simulink library "INP_DMP_ManOver"  (R2024b)
settings: Solver=VariableStepAuto  StartTime=0.0  StopTime=10.0  RelTol=1e-3
undefined symbols (not defined in the file): INP_DMP_p_StrkDmpLoLimFrLe_mm, INP_DMP_p_StrkDmpLoLimFrRi_mm, INP_DMP_p_StrkDmpLoLimReLe_mm, INP_DMP_p_StrkDmpLoLimReRi_mm, INP_DMP_p_StrkDmpUpLimFrLe_mm, INP_DMP_p_StrkDmpUpLimFrRi_mm, INP_DMP_p_StrkDmpUpLimReLe_mm, INP_DMP_p_StrkDmpUpLimReRi_mm, INP_DMP_p_SwtStrkDmpFrLe_na, INP_DMP_p_SwtStrkDmpFrRi_na, INP_DMP_p_SwtStrkDmpReLe_na, INP_DMP_p_SwtStrkDmpReRi_na, INP_DMP_s_StrkDmpFrLeMan_mm, INP_DMP_s_StrkDmpFrRiMan_mm, INP_DMP_s_StrkDmpReLeMan_mm, INP_DMP_s_StrkDmpReRiMan_mm, INP_DRVR_p_AngRatStWhlLoLim_radps, INP_DRVR_p_AngRatStWhlUpLim_radps, INP_DRVR_p_AngStWhlLoLim_rad, INP_DRVR_p_AngStWhlUpLim_rad, INP_DRVR_p_PosRatThrLoLim_p100ps, INP_DRVR_p_PosRatThrMan_p100ps, INP_DRVR_p_PosRatThrUpLim_p100ps, INP_DRVR_p_PosThrLoLim_p100, INP_DRVR_p_PosThrMan_p100, INP_DRVR_p_PosThrUpLim_p100, INP_DRVR_p_SwtAngRatStWhlMan_na, INP_DRVR_p_SwtAngStWhlMan_na, INP_DRVR_p_SwtPosRatThrMan_na, INP_DRVR_p_SwtPosThrMan_na, INP_DRVR_s_AngRatStWhlMan_radps, INP_DRVR_s_AngStWhlMan_rad
libraries: simulink x8
settings Model: Creator=blatak  LastModifiedBy=jmbsp

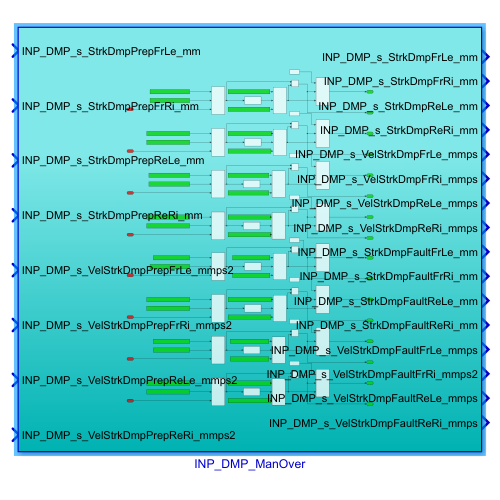
[thumbnail: Simulink's stored preview of the top-level diagram]
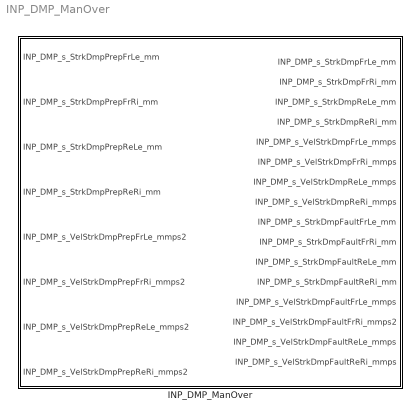
== system INP_DMP_ManOver ==
  INP_DMP_ManOver : Subsystem

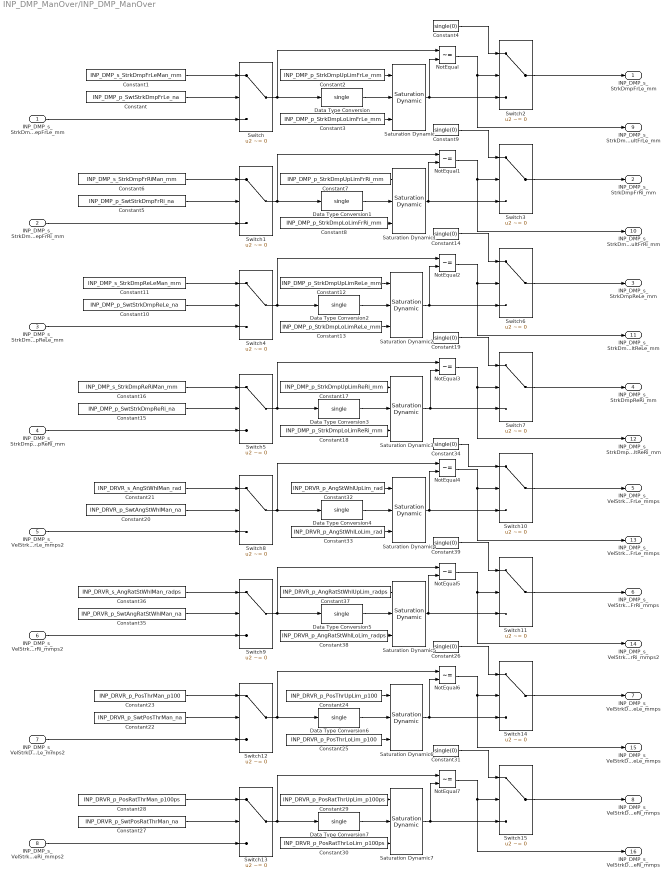
== system INP_DMP_ManOver/INP_DMP_ManOver ==
  INP_DMP_s_StrkDmpPrepFrLe_mm : Inport
  INP_DMP_s_StrkDmpPrepFrRi_mm : Inport  Port=2
  INP_DMP_s_StrkDmpPrepReLe_mm : Inport  Port=3
  INP_DMP_s_StrkDmpPrepReRi_mm : Inport  Port=4
  INP_DMP_s_VelStrkDmpPrepFrLe_mmps2 : Inport  Port=5
  INP_DMP_s_VelStrkDmpPrepFrRi_mmps2 : Inport  Port=6
  INP_DMP_s_VelStrkDmpPrepReLe_mmps2 : Inport  Port=7
  INP_DMP_s_VelStrkDmpPrepReRi_mmps2 : Inport  Port=8
  Constant : Constant  Description=|  Value=INP_DMP_p_SwtStrkDmpFrLe_na
      | Switch for manual override of the longitudinal acceleration value, if 1 instead the measured 
      | value the INP_IMU_p_ALgtVehMan_mps2 is used
  Constant1 : Constant  Description=|  Value=INP_DMP_s_StrkDmpFrLeMan_mm
      | Value for longitudinal acceleration, which is used if the INP_IMU_p_SwtAXxxVehMan_na
      | is set to 1 instead of the measured value
  Constant10 : Constant  Description=|  Value=INP_DMP_p_SwtStrkDmpReLe_na
      | Switch for manual override of the longitudinal acceleration value, if 1 instead the measured 
      | value the INP_IMU_p_ALgtVehMan_mps2 is used
  Constant11 : Constant  Description=|  Value=INP_DMP_s_StrkDmpReLeMan_mm
      | Value for longitudinal acceleration, which is used if the INP_IMU_p_SwtAXxxVehMan_na
      | is set to 1 instead of the measured value
  Constant12 : Constant  Description=Upper saturation limit for longitudinal acceleration  Value=INP_DMP_p_StrkDmpUpLimReLe_mm
  Constant13 : Constant  Description=Lower saturation limit for longitudinal acceleration  Value=INP_DMP_p_StrkDmpLoLimReLe_mm
  Constant{4,9,14,19,26,31,34,39} (8 alike) : Constant  Value=single(0)
  Constant15 : Constant  Description=|  Value=INP_DMP_p_SwtStrkDmpReRi_na
      | Switch for manual override of the longitudinal acceleration value, if 1 instead the measured 
      | value the INP_IMU_p_ALgtVehMan_mps2 is used
  Constant16 : Constant  Description=|  Value=INP_DMP_s_StrkDmpReRiMan_mm
      | Value for longitudinal acceleration, which is used if the INP_IMU_p_SwtAXxxVehMan_na
      | is set to 1 instead of the measured value
  Constant17 : Constant  Description=Upper saturation limit for longitudinal acceleration  Value=INP_DMP_p_StrkDmpUpLimReRi_mm
  Constant18 : Constant  Description=Lower saturation limit for longitudinal acceleration  Value=INP_DMP_p_StrkDmpLoLimReRi_mm
  Constant2 : Constant  Description=Upper saturation limit for longitudinal acceleration  Value=INP_DMP_p_StrkDmpUpLimFrLe_mm
  Constant20 : Constant  Description=|  Value=INP_DRVR_p_SwtAngStWhlMan_na
      | Switch for manual override of the longitudinal acceleration value, if 1 instead the measured 
      | value the INP_IMU_p_ALgtVehMan_mps2 is used
  Constant21 : Constant  Description=|  Value=INP_DRVR_s_AngStWhlMan_rad
      | Value for longitudinal acceleration, which is used if the INP_IMU_p_SwtAXxxVehMan_na
      | is set to 1 instead of the measured value
  Constant22 : Constant  Description=|  Value=INP_DRVR_p_SwtPosThrMan_na
      | Switch for manual override of the longitudinal acceleration value, if 1 instead the measured 
      | value the INP_IMU_p_ALgtVehMan_mps2 is used
  Constant23 : Constant  Description=|  Value=INP_DRVR_p_PosThrMan_p100
      | Value for longitudinal acceleration, which is used if the INP_IMU_p_SwtAXxxVehMan_na
      | is set to 1 instead of the measured value
  Constant24 : Constant  Description=Upper saturation limit for longitudinal acceleration  Value=INP_DRVR_p_PosThrUpLim_p100
  Constant25 : Constant  Description=Lower saturation limit for longitudinal acceleration  Value=INP_DRVR_p_PosThrLoLim_p100
  Constant27 : Constant  Description=|  Value=INP_DRVR_p_SwtPosRatThrMan_na
      | Switch for manual override of the longitudinal acceleration value, if 1 instead the measured 
      | value the INP_IMU_p_ALgtVehMan_mps2 is used
  Constant28 : Constant  Description=|  Value=INP_DRVR_p_PosRatThrMan_p100ps
      | Value for longitudinal acceleration, which is used if the INP_IMU_p_SwtAXxxVehMan_na
      | is set to 1 instead of the measured value
  Constant29 : Constant  Description=Upper saturation limit for longitudinal acceleration  Value=INP_DRVR_p_PosRatThrUpLim_p100ps
  Constant3 : Constant  Description=Lower saturation limit for longitudinal acceleration  Value=INP_DMP_p_StrkDmpLoLimFrLe_mm
  Constant30 : Constant  Description=Lower saturation limit for longitudinal acceleration  Value=INP_DRVR_p_PosRatThrLoLim_p100ps
  Constant32 : Constant  Description=Upper saturation limit for longitudinal acceleration  Value=INP_DRVR_p_AngStWhlUpLim_rad
  Constant33 : Constant  Description=Lower saturation limit for longitudinal acceleration  Value=INP_DRVR_p_AngStWhlLoLim_rad
  Constant35 : Constant  Description=|  Value=INP_DRVR_p_SwtAngRatStWhlMan_na
      | Switch for manual override of the longitudinal acceleration value, if 1 instead the measured 
      | value the INP_IMU_p_ALgtVehMan_mps2 is used
  Constant36 : Constant  Description=|  Value=INP_DRVR_s_AngRatStWhlMan_radps
      | Value for longitudinal acceleration, which is used if the INP_IMU_p_SwtAXxxVehMan_na
      | is set to 1 instead of the measured value
  Constant37 : Constant  Description=Upper saturation limit for longitudinal acceleration  Value=INP_DRVR_p_AngRatStWhlUpLim_radps
  Constant38 : Constant  Description=Lower saturation limit for longitudinal acceleration  Value=INP_DRVR_p_AngRatStWhlLoLim_radps
  Constant5 : Constant  Description=|  Value=INP_DMP_p_SwtStrkDmpFrRi_na
      | Switch for manual override of the longitudinal acceleration value, if 1 instead the measured 
      | value the INP_IMU_p_ALgtVehMan_mps2 is used
  Constant6 : Constant  Description=|  Value=INP_DMP_s_StrkDmpFrRiMan_mm
      | Value for longitudinal acceleration, which is used if the INP_IMU_p_SwtAXxxVehMan_na
      | is set to 1 instead of the measured value
  Constant7 : Constant  Description=Upper saturation limit for longitudinal acceleration  Value=INP_DMP_p_StrkDmpUpLimFrRi_mm
  Constant8 : Constant  Description=Lower saturation limit for longitudinal acceleration  Value=INP_DMP_p_StrkDmpLoLimFrRi_mm
  Data Type Conversion{,1..7} (8 alike) : DataTypeConversion  OutDataTypeStr=single  SaturateOnIntegerOverflow=off  RndMeth=Floor
  NotEqual{,1..7} (8 alike) : RelationalOperator  Operator=~=  OutDataTypeStr=boolean  RndMeth=Simplest  InputSameDT=off
  Saturation Dynamic{,1..7} (8 alike) : simulink/Discontinuities/Saturation Dynamic  OutMin=[]  OutMax=[]  OutDataTypeStr=Inherit: Same as second input  OutDataType=fixdt(1, 16)  OutScaling=2^-10  DoSatur=off
  Switch{,1..15} (16 alike) : Switch  Criteria=u2 ~= 0  SaturateOnIntegerOverflow=off  InputSameDT=off
  INP_DMP_s_StrkDmpFrLe_mm : Outport
  INP_DMP_s_StrkDmpFrRi_mm : Outport  Port=2
  INP_DMP_s_StrkDmpReLe_mm : Outport  Port=3
  INP_DMP_s_StrkDmpReRi_mm : Outport  Port=4
  INP_DMP_s_VelStrkDmpFrLe_mmps : Outport  Port=5
  INP_DMP_s_VelStrkDmpFrRi_mmps : Outport  Port=6
  INP_DMP_s_VelStrkDmpReLe_mmps : Outport  Port=7
  INP_DMP_s_VelStrkDmpReRi_mmps : Outport  Port=8
  INP_DMP_s_StrkDmpFaultFrLe_mm : Outport  Port=9
  INP_DMP_s_StrkDmpFaultFrRi_mm : Outport  Port=10
  INP_DMP_s_StrkDmpFaultReLe_mm : Outport  Port=11
  INP_DMP_s_StrkDmpFaultReRi_mm : Outport  Port=12
  INP_DMP_s_VelStrkDmpFaultFrLe_mmps : Outport  Port=13
  INP_DMP_s_VelStrkDmpFaultFrRi_mmps2 : Outport  Port=14
  INP_DMP_s_VelStrkDmpFaultReLe_mmps : Outport  Port=15
  INP_DMP_s_VelStrkDmpFaultReRi_mmps : Outport  Port=16
  wires:
  Switch/1 -> NotEqual/1, Data Type Conversion/1
  NotEqual2/1 -> INP_DMP_s_StrkDmpFaultReLe_mm/1, Switch6/2
  Saturation Dynamic1/1 -> Switch3/3, NotEqual1/2
  Constant16/1 -> Switch5/1
  Constant11/1 -> Switch4/1
  Switch4/1 -> NotEqual2/1, Data Type Conversion2/1
  Switch1/1 -> NotEqual1/1, Data Type Conversion1/1
  Constant7/1 -> Saturation Dynamic1/1
  Constant2/1 -> Saturation Dynamic/1
  Constant/1 -> Switch/2
  Data Type Conversion/1 -> Saturation Dynamic/2
  Constant12/1 -> Saturation Dynamic2/1
  INP_DMP_s_StrkDmpPrepReRi_mm/1 -> Switch5/3
  Switch7/1 -> INP_DMP_s_StrkDmpReRi_mm/1
  Saturation Dynamic3/1 -> Switch7/3, NotEqual3/2
  Switch5/1 -> NotEqual3/1, Data Type Conversion3/1
  Constant6/1 -> Switch1/1
  NotEqual3/1 -> INP_DMP_s_StrkDmpFaultReRi_mm/1, Switch7/2
  Data Type Conversion2/1 -> Saturation Dynamic2/2
  INP_DMP_s_StrkDmpPrepFrRi_mm/1 -> Switch1/3
  Constant17/1 -> Saturation Dynamic3/1
  NotEqual/1 -> INP_DMP_s_StrkDmpFaultFrLe_mm/1, Switch2/2
  Constant15/1 -> Switch5/2
  Saturation Dynamic2/1 -> Switch6/3, NotEqual2/2
  Data Type Conversion3/1 -> Saturation Dynamic3/2
  Constant9/1 -> Switch3/1
  Switch6/1 -> INP_DMP_s_StrkDmpReLe_mm/1
  Data Type Conversion1/1 -> Saturation Dynamic1/2
  Constant3/1 -> Saturation Dynamic/3
  Saturation Dynamic/1 -> Switch2/3, NotEqual/2
  Constant1/1 -> Switch/1
  Constant8/1 -> Saturation Dynamic1/3
  NotEqual1/1 -> INP_DMP_s_StrkDmpFaultFrRi_mm/1, Switch3/2
  Constant18/1 -> Saturation Dynamic3/3
  Constant13/1 -> Saturation Dynamic2/3
  Constant5/1 -> Switch1/2
  Constant19/1 -> Switch7/1
  Switch2/1 -> INP_DMP_s_StrkDmpFrLe_mm/1
  INP_DMP_s_StrkDmpPrepFrLe_mm/1 -> Switch/3
  Constant4/1 -> Switch2/1
  INP_DMP_s_StrkDmpPrepReLe_mm/1 -> Switch4/3
  Constant10/1 -> Switch4/2
  Constant14/1 -> Switch6/1
  Switch3/1 -> INP_DMP_s_StrkDmpFrRi_mm/1
  Constant29/1 -> Saturation Dynamic7/1
  Constant25/1 -> Saturation Dynamic6/3
  Data Type Conversion6/1 -> Saturation Dynamic6/2
  Constant35/1 -> Switch9/2
  INP_DMP_s_VelStrkDmpPrepFrRi_mmps2/1 -> Switch9/3
  Constant39/1 -> Switch11/1
  Constant20/1 -> Switch8/2
  Saturation Dynamic5/1 -> Switch11/3, NotEqual5/2
  Constant31/1 -> Switch15/1
  Constant26/1 -> Switch14/1
  INP_DMP_s_VelStrkDmpPrepFrLe_mmps2/1 -> Switch8/3
  Constant24/1 -> Saturation Dynamic6/1
  NotEqual5/1 -> INP_DMP_s_VelStrkDmpFaultFrRi_mmps2/1, Switch11/2
  Data Type Conversion7/1 -> Saturation Dynamic7/2
  Constant28/1 -> Switch13/1
  Saturation Dynamic4/1 -> Switch10/3, NotEqual4/2
  Data Type Conversion4/1 -> Saturation Dynamic4/2
  Constant38/1 -> Saturation Dynamic5/3
  Constant23/1 -> Switch12/1
  Constant22/1 -> Switch12/2
  Constant32/1 -> Saturation Dynamic4/1
  NotEqual7/1 -> INP_DMP_s_VelStrkDmpFaultReRi_mmps/1, Switch15/2
  Switch9/1 -> NotEqual5/1, Data Type Conversion5/1
  Switch11/1 -> INP_DMP_s_VelStrkDmpFrRi_mmps/1
  Saturation Dynamic6/1 -> Switch14/3, NotEqual6/2
  Switch15/1 -> INP_DMP_s_VelStrkDmpReRi_mmps/1
  Constant30/1 -> Saturation Dynamic7/3
  INP_DMP_s_VelStrkDmpPrepReRi_mmps2/1 -> Switch13/3
  Switch12/1 -> NotEqual6/1, Data Type Conversion6/1
  Constant33/1 -> Saturation Dynamic4/3
  Switch14/1 -> INP_DMP_s_VelStrkDmpReLe_mmps/1
  INP_DMP_s_VelStrkDmpPrepReLe_mmps2/1 -> Switch12/3
  NotEqual4/1 -> INP_DMP_s_VelStrkDmpFaultFrLe_mmps/1, Switch10/2
  Switch8/1 -> NotEqual4/1, Data Type Conversion4/1
  Switch10/1 -> INP_DMP_s_VelStrkDmpFrLe_mmps/1
  Constant21/1 -> Switch8/1
  Constant36/1 -> Switch9/1
  Constant34/1 -> Switch10/1
  Switch13/1 -> NotEqual7/1, Data Type Conversion7/1
  Data Type Conversion5/1 -> Saturation Dynamic5/2
  Saturation Dynamic7/1 -> Switch15/3, NotEqual7/2
  Constant27/1 -> Switch13/2
  NotEqual6/1 -> INP_DMP_s_VelStrkDmpFaultReLe_mmps/1, Switch14/2
  Constant37/1 -> Saturation Dynamic5/1
